simulink library "null_allocation_lib"  (R2018b)
settings: Solver=VariableStepAuto  StartTime=0.0  StopTime=10.0  RelTol=1e-3
undefined symbols (not defined in the file or in its folder): fswParams
settings Model: Creator=Nick's PC  LastModifiedBy=Nick's PC

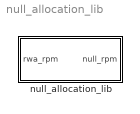
== system null_allocation_lib ==
  null_allocation_lib : Subsystem

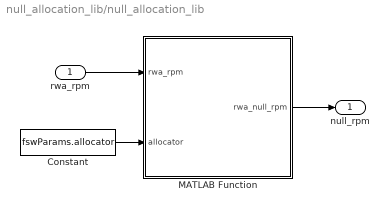
== system null_allocation_lib/null_allocation_lib ==
  rwa_rpm : Inport
  Constant : Constant  Value=fswParams.allocator  OutDataTypeStr=Bus: RWA
  MATLAB Function : MATLAB Function  TreatAsAtomicUnit=on
  null_rpm : Outport
  wires:
  rwa_rpm/1 -> MATLAB Function/1(rwa_rpm)
  MATLAB Function/1(rwa_null_rpm) -> null_rpm/1
  Constant/1 -> MATLAB Function/2(allocator)

== matlab function null_allocation_lib/MATLAB Function ==
  data: rwa_rpm input; rwa_null_rpm output; allocator input
function rwa_null_rpm = alloc_null(rwa_rpm,allocator)
%#codegen
RPM2RPS = 2*pi()/60;

RPS2RPM = 60/(2*pi());

h_targ = allocator.h_targ_wheel_Nms;

nullvec = allocator.rwa_nullvec;

h_rwa = rwa_rpm .* RPM2RPS .* allocator.inertia;

h_err = h_targ - h_rwa;

h_err_null_norm = h_err ./ nullvec;

rw_max = max(h_err_null_norm);

rw_min = min(h_err_null_norm);

null_multiplier = (rw_max + rw_min)/2;

rwa_optimal_null_Nm = -null_multiplier*nullvec;

rwa_null_rpm = (rwa_optimal_null_Nm ./ allocator.inertia) .* RPS2RPM;

end
